simulink model "Ugorny_lab5s"  (R2020b)
settings: Solver=VariableStepAuto  StartTime=0.0  StopTime=10.0  RelTol=1e-3
values from neighbouring files (symbols this model uses):
  du = 1    [Ugorny_lab5.m]
  Ksi = KsiList(j,i)    [Ugorny_lab5.m]
  t0 = 0    [Ugorny_lab5.m]
  u0 = 0    [Ugorny_lab5.m]
  Wn = WnList(j,i)    [Ugorny_lab5.m]
settings Model: Creator=Lab320  LastModifiedBy=Lab320

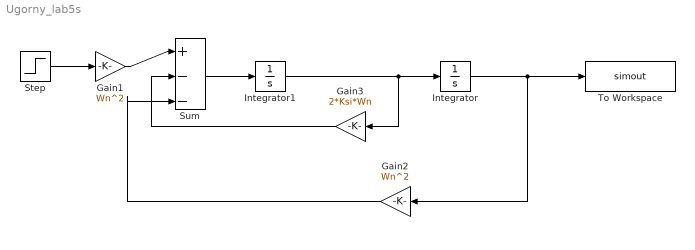
== system Ugorny_lab5s ==
  Gain1 : Gain  Gain=Wn^2
  Gain2 : Gain  Gain=Wn^2
  Gain3 : Gain  Gain=2*Ksi*Wn
  Integrator : Integrator
  Integrator1 : Integrator
  Step : Step  Time=t0  Before=u0  After=u0 + du  SampleTime=0
  Sum : Sum  Inputs=|+--
  To Workspace : ToWorkspace  VariableName=simout  SampleTime=-1
  wires:
  Step/1 -> Gain1/1
  Sum/1 -> Integrator1/1
  Integrator1/1 -> Gain3/1, Integrator/1
  Gain3/1 -> Sum/2
  Integrator/1 -> Gain2/1, To Workspace/1
  Gain2/1 -> Sum/3
  Gain1/1 -> Sum/1
